simulink model "L0203"  (Simulink 10.2)
settings: Solver=ode45  StartTime=0.0  StopTime=20  MaxStep=0.01  RelTol=1e-3
model workspace (MAT data in the model file):
  x0 : num (value not decoded)
settings Model: Creator=Ranci  LastModifiedBy=Ranci
settings DataIOCC: SaveFormat=Dataset  SignalLoggingSaveFormat=Dataset  ReturnWorkspaceOutputs=on
settings OptimizationCC: LifeSpan=auto
settings DebuggingCC: UnderspecifiedInitializationDetection=Simplified  MergeDetectMultiDrivingBlocksExec=error  FcnCallInpInsideContextMsg=error  SFUnexpectedBacktrackingDiag=error  SFNoUnconditionalDefaultTransitionDiag=error  SFExecutionAtInitializationDiag=warning  ArithmeticOperatorsInVariantConditions=error
settings HardwareCC: ProdBitPerPointer=64  ProdBitPerSizeT=64  ProdBitPerPtrDiffT=64  ProdLargestAtomicFloat=Float  ProdIntDivRoundTo=Zero  ProdEndianess=LittleEndian  ProdWordSize=64  ProdHWDeviceType=Intel->x86-64 (Windows64)
settings ModelReferenceCC: PropagateSignalLabelsOutOfModel=on
settings SFSimCC: SimUseLocalCustomCode=on  CustomCodeUndefinedFunction=FilterOut
settings RTWCC: RTWUseLocalCustomCode=on
settings CodeAppCC: StateflowObjectComments=off
settings GRTTargetCC: TargetLangStandard=C99 (ISO)  CombineOutputUpdateFcns=on  GRTInterface=off
settings ConfigComp: CovMetricSettings=dwe  CovSaveCumulativeToWorkspaceVar=off  CovSaveSingleToWorkspaceVar=off  CovExternalEMLEnable=on

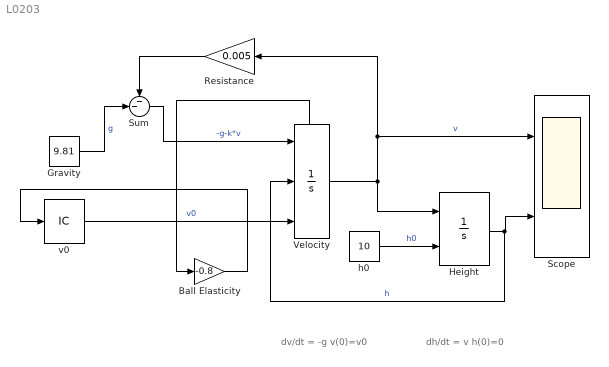
== system L0203 ==
  note: dv/dt = -g
      | v(0)=v0
  note: dh/dt = v
      | h(0)=0
  Ball Elasticity : Gain  Gain=-0.8
  Gravity : Constant  Value=9.81
  Height : Integrator  InitialConditionSource=external  LimitOutput=on  LowerSaturationLimit=0
  Resistance : Gain  Gain=0.005
  Scope : Scope  NumInputPorts=2
  Sum : Sum  Inputs=--|
  Velocity : Integrator  ExternalReset=falling  InitialConditionSource=external  ShowStatePort=on
  h0 : Constant  Value=10
  v0 : InitialCondition  Value=15
  wires:
  Sum/1 -> Velocity/1  "-g-k*v"
  Velocity/1 -> Resistance/1, Scope/1, Height/1  "v"
  Height/1 -> Velocity/2, Scope/2  "h"
  h0/1 -> Height/2  "h0"
  v0/1 -> Velocity/3  "v0"
  Velocity/State -> Ball Elasticity/1
  Ball Elasticity/1 -> v0/1
  Gravity/1 -> Sum/2  "g"
  Resistance/1 -> Sum/1
